simulink model "YAw_sim"  (R2018b)
settings: Solver=VariableStepAuto  StartTime=0.0  StopTime=10.0  RelTol=1e-3
settings Model: Creator=a4327  LastModifiedBy=a4327

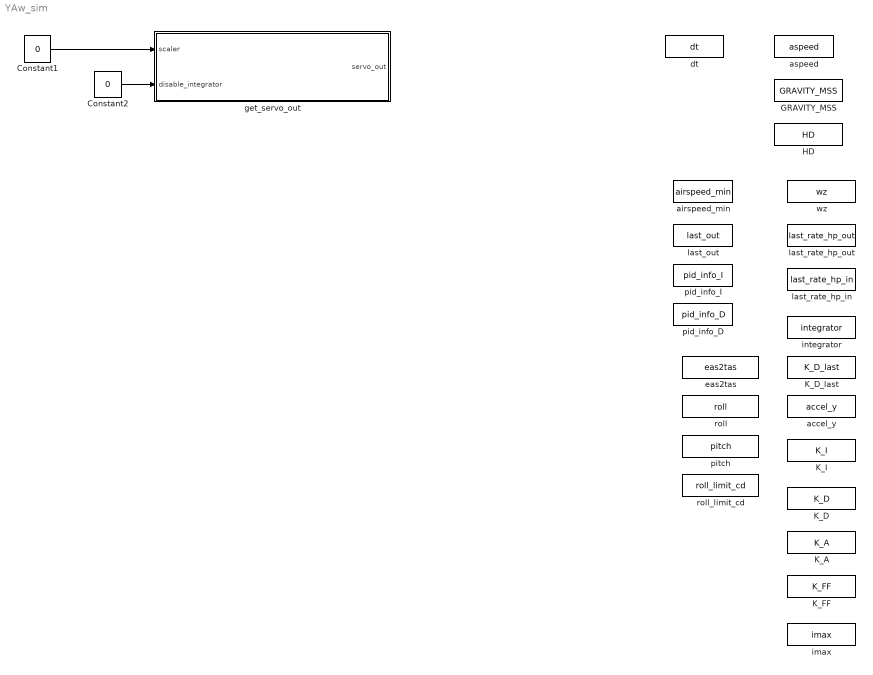
== system YAw_sim ==
  Constant1 : Constant  Value=0
  Constant2 : Constant  Value=0
  GRAVITY_MSS : DataStoreMemory  DataStoreName=GRAVITY_MSS  ReadBeforeWriteMsg=warning  WriteAfterWriteMsg=warning  WriteAfterReadMsg=warning  InitialValue=GRAVITY_MSS  ShowAdditionalParam=off  OutDataTypeStr=double
  HD : DataStoreMemory  DataStoreName=HD  ReadBeforeWriteMsg=warning  WriteAfterWriteMsg=warning  WriteAfterReadMsg=warning  InitialValue=HD  ShowAdditionalParam=off  OutDataTypeStr=double
  K_A : DataStoreMemory  DataStoreName=K_A  ReadBeforeWriteMsg=warning  WriteAfterWriteMsg=warning  WriteAfterReadMsg=warning  InitialValue=K_A  ShowAdditionalParam=off  OutDataTypeStr=double
  K_D : DataStoreMemory  DataStoreName=K_D  ReadBeforeWriteMsg=warning  WriteAfterWriteMsg=warning  WriteAfterReadMsg=warning  InitialValue=K_D  ShowAdditionalParam=off  OutDataTypeStr=double
  K_D_last : DataStoreMemory  DataStoreName=K_D_last  ReadBeforeWriteMsg=warning  WriteAfterWriteMsg=warning  WriteAfterReadMsg=warning  InitialValue=K_D_last  ShowAdditionalParam=off  OutDataTypeStr=double
  K_FF : DataStoreMemory  DataStoreName=K_FF  ReadBeforeWriteMsg=warning  WriteAfterWriteMsg=warning  WriteAfterReadMsg=warning  InitialValue=K_FF  ShowAdditionalParam=off  OutDataTypeStr=double
  K_I : DataStoreMemory  DataStoreName=K_I  ReadBeforeWriteMsg=warning  WriteAfterWriteMsg=warning  WriteAfterReadMsg=warning  InitialValue=K_I  ShowAdditionalParam=off  OutDataTypeStr=double
  accel_y : DataStoreMemory  DataStoreName=accel_y  ReadBeforeWriteMsg=warning  WriteAfterWriteMsg=warning  WriteAfterReadMsg=warning  InitialValue=accel_y  ShowAdditionalParam=off  OutDataTypeStr=double
  airspeed_min : DataStoreMemory  DataStoreName=airspeed_min  ReadBeforeWriteMsg=warning  WriteAfterWriteMsg=warning  WriteAfterReadMsg=warning  InitialValue=airspeed_min  ShowAdditionalParam=off  OutDataTypeStr=double
  aspeed : DataStoreMemory  DataStoreName=aspeed  ReadBeforeWriteMsg=warning  WriteAfterWriteMsg=warning  WriteAfterReadMsg=warning  InitialValue=aspeed  ShowAdditionalParam=off  OutDataTypeStr=double
  dt : DataStoreMemory  DataStoreName=dt  ReadBeforeWriteMsg=warning  WriteAfterWriteMsg=warning  WriteAfterReadMsg=warning  InitialValue=dt  ShowAdditionalParam=off  OutDataTypeStr=double
  eas2tas : DataStoreMemory  DataStoreName=eas2tas  ReadBeforeWriteMsg=warning  WriteAfterWriteMsg=warning  WriteAfterReadMsg=warning  InitialValue=eas2tas  ShowAdditionalParam=off  OutDataTypeStr=double
  get_servo_out : MATLAB Function  TreatAsAtomicUnit=on
  imax : DataStoreMemory  DataStoreName=imax  ReadBeforeWriteMsg=warning  WriteAfterWriteMsg=warning  WriteAfterReadMsg=warning  InitialValue=imax  ShowAdditionalParam=off  OutDataTypeStr=double
  integrator : DataStoreMemory  DataStoreName=integrator  ReadBeforeWriteMsg=warning  WriteAfterWriteMsg=warning  WriteAfterReadMsg=warning  InitialValue=integrator  ShowAdditionalParam=off  OutDataTypeStr=double
  last_out : DataStoreMemory  DataStoreName=last_out  ReadBeforeWriteMsg=warning  WriteAfterWriteMsg=warning  WriteAfterReadMsg=warning  InitialValue=last_out  ShowAdditionalParam=off  OutDataTypeStr=double
  last_rate_hp_in : DataStoreMemory  DataStoreName=last_rate_hp_in  ReadBeforeWriteMsg=warning  WriteAfterWriteMsg=warning  WriteAfterReadMsg=warning  InitialValue=last_rate_hp_in  ShowAdditionalParam=off  OutDataTypeStr=double
  last_rate_hp_out : DataStoreMemory  DataStoreName=last_rate_hp_out  ReadBeforeWriteMsg=warning  WriteAfterWriteMsg=warning  WriteAfterReadMsg=warning  InitialValue=last_rate_hp_out  ShowAdditionalParam=off  OutDataTypeStr=double
  pid_info_D : DataStoreMemory  DataStoreName=pid_info_D  ReadBeforeWriteMsg=warning  WriteAfterWriteMsg=warning  WriteAfterReadMsg=warning  InitialValue=pid_info_D  ShowAdditionalParam=off  OutDataTypeStr=double
  pid_info_I : DataStoreMemory  DataStoreName=pid_info_I  ReadBeforeWriteMsg=warning  WriteAfterWriteMsg=warning  WriteAfterReadMsg=warning  InitialValue=pid_info_I  ShowAdditionalParam=off  OutDataTypeStr=double
  pitch : DataStoreMemory  DataStoreName=pitch  ReadBeforeWriteMsg=warning  WriteAfterWriteMsg=warning  WriteAfterReadMsg=warning  InitialValue=pitch  ShowAdditionalParam=off  OutDataTypeStr=double
  roll : DataStoreMemory  DataStoreName=roll  ReadBeforeWriteMsg=warning  WriteAfterWriteMsg=warning  WriteAfterReadMsg=warning  InitialValue=roll  ShowAdditionalParam=off  OutDataTypeStr=double
  roll_limit_cd : DataStoreMemory  DataStoreName=roll_limit_cd  ReadBeforeWriteMsg=warning  WriteAfterWriteMsg=warning  WriteAfterReadMsg=warning  InitialValue=roll_limit_cd  ShowAdditionalParam=off  OutDataTypeStr=double
  wz : DataStoreMemory  DataStoreName=wz  ReadBeforeWriteMsg=warning  WriteAfterWriteMsg=warning  WriteAfterReadMsg=warning  InitialValue=wz  ShowAdditionalParam=off  OutDataTypeStr=double
  wires:
  Constant1/1 -> get_servo_out/1(scaler)
  Constant2/1 -> get_servo_out/2(disable_integrator)

== matlab function YAw_sim/get_servo_out ==
  data: servo_out output; scaler input; disable_integrator input; dt data_store_memory; airspeed_min data_store_memory; last_out data_store_memory; pid_info_I data_store_memory; pid_info_D data_store_memory; eas2tas data_store_memory; roll data_store_memory; pitch data_store_memory; roll_limit_cd data_store_memory; aspeed data_store_memory; GRAVITY_MSS data_store_memory; HD data_store_memory; wz data_store_memory; last_rate_hp_out data_store_memory; last_rate_hp_in data_store_memory; integrator data_store_memory; K_D_last data_store_memory; accel_y data_store_memory; K_I data_store_memory; K_D data_store_memory; K_A data_store_memory; K_FF data_store_memory; imax data_store_memory
function servo_out=get_servo_out(  scaler,   disable_integrator)

servo_out=get_servo_out(  scaler,   disable_integrator);
